simulink model "two_area_model_P_control"  (R2014b)
settings: Solver=ode4  StartTime=0.0  StopTime=10.0  FixedStep=0.01  RelTol=1e-3
settings Model: Creator=Shane Reynolds  LastModifiedBy=Shane Reynolds

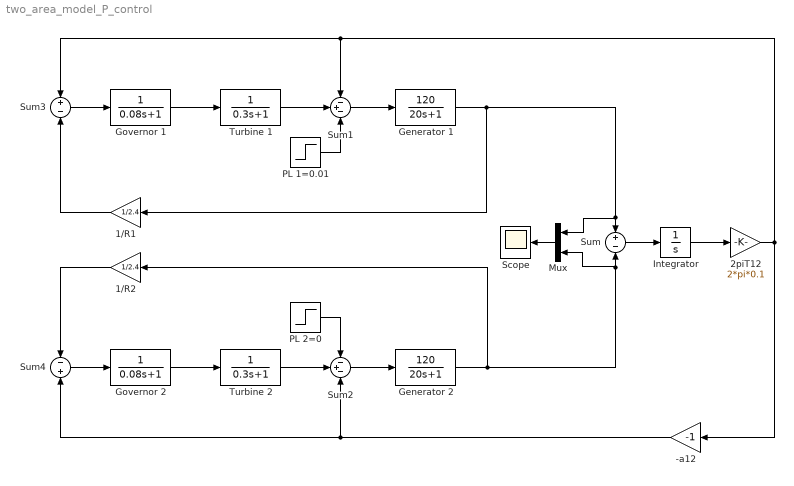
== system two_area_model_P_control ==
  -a12 : Gain  Gain=-1
  1/R1 : Gain  Gain=1/2.4
  1/R2 : Gain  Gain=1/2.4
  2piT12 : Gain  Gain=2*pi*0.1
  Generator 1 : TransferFcn  Numerator=[120]  Denominator=[20 1]
  Generator 2 : TransferFcn  Numerator=[120]  Denominator=[20 1]
  Governor 1 : TransferFcn  Denominator=[0.08 1]
  Governor 2 : TransferFcn  Denominator=[0.08 1]
  Integrator : Integrator
  Mux : Mux  Inputs=2
  PL 1=0.01 : Step  After=0.01  SampleTime=0
  PL 2=0 : Step  After=0  SampleTime=0
  Scope : Scope
  Sum : Sum  Inputs=+|-
  Sum1 : Sum  Inputs=-+-
  Sum2 : Sum  Inputs=-+-
  Sum3 : Sum  Inputs=+|-
  Sum4 : Sum  Inputs=-|+
  Turbine 1 : TransferFcn  Denominator=[0.3 1]
  Turbine 2 : TransferFcn  Denominator=[0.3 1]
  wires:
  Turbine 1/1 -> Sum1/2
  Sum1/1 -> Generator 1/1
  Turbine 2/1 -> Sum2/2
  Sum2/1 -> Generator 2/1
  Governor 1/1 -> Turbine 1/1
  Governor 2/1 -> Turbine 2/1
  Sum4/1 -> Governor 2/1
  Sum3/1 -> Governor 1/1
  Generator 1/1 -> 1/R1/1, Mux/1, Sum/1
  Generator 2/1 -> 1/R2/1, Mux/2, Sum/2
  Sum/1 -> Integrator/1
  Integrator/1 -> 2piT12/1
  1/R1/1 -> Sum3/2
  1/R2/1 -> Sum4/1
  2piT12/1 -> Sum1/1, Sum3/1, -a12/1
  -a12/1 -> Sum2/3, Sum4/2
  Mux/1 -> Scope/1
  PL 1=0.01/1 -> Sum1/3
  PL 2=0/1 -> Sum2/1
